simulink model "prve"  (Simulink 7.9)
settings: Solver=ode3  StartTime=0.0  StopTime=t_sim  RelTol=1e-3
values from neighbouring files (symbols this model uses):
  baud = 250000    [init.m]    (also in init_101_io_char_up_oloop.m)
  bulb = 100    [init.m]
  com = 'COM8'    [init.m]    (also in init_101_io_char_up_oloop.m = 'COM33')
  fan = 0    [init.m]
  fTf = 0.2    [init.m]    (also in init_101_io_char_up_oloop.m)
  fTl = 0.2    [init.m]    (also in init_101_io_char_up_oloop.m)
  fTt = 0.2    [init.m]    (also in init_101_io_char_up_oloop.m)
  LED = 0    [init.m]
  Ts = 0.1    [init.m]    (also in init_101_io_char_up_oloop.m)
libraries: tos_lib x1
settings Model: Creator=tom  LastModifiedBy=Katka
settings DataIOCC: LimitDataPoints=off
settings DebuggingCC: FcnCallInpInsideContextMsg=Use local settings  StrictBusMsg=Warning
settings GRTTargetCC: CombineOutputUpdateFcns=off  GRTInterface=on

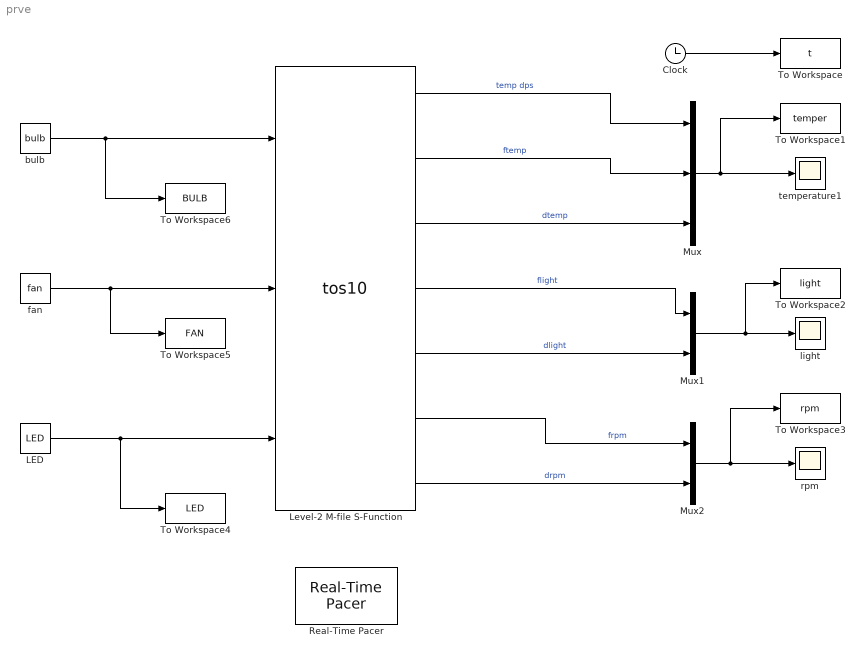
== system prve ==
  Clock : Clock
  LED : Constant  Value=LED
  Level-2 M-file S-Function : M-S-Function  FunctionName=tos10  Parameters=Ts,com,baud,fTt,fTl,fTf
  Mux : Mux  Inputs=3
  Mux1 : Mux  Inputs=2
  Mux2 : Mux  Inputs=2
  Real-Time Pacer : tos_lib/Real-Time Pacer  simTimePerRealTime=1
  To Workspace : ToWorkspace  VariableName=t  SampleTime=Ts
  To Workspace1 : ToWorkspace  VariableName=temper  SampleTime=Ts
  To Workspace2 : ToWorkspace  VariableName=light  SampleTime=Ts
  To Workspace3 : ToWorkspace  VariableName=rpm  SampleTime=Ts
  To Workspace4 : ToWorkspace  VariableName=LED  SampleTime=Ts
  To Workspace5 : ToWorkspace  VariableName=FAN  SampleTime=Ts
  To Workspace6 : ToWorkspace  VariableName=BULB  SampleTime=Ts
  bulb : Constant  Value=bulb
  fan : Constant  Value=fan
  light : Scope
      settings: YMax=85  MaxDataPoints=50000
  rpm : Scope
      settings: YMax=85  MaxDataPoints=50000
  temperature1 : Scope
      settings: TimeRange=2400  YMin=-2.5  YMax=45  SaveName=ScopeData4  MaxDataPoints=50000
  wires:
  bulb/1 -> Level-2 M-file S-Function/1, To Workspace6/1
  fan/1 -> Level-2 M-file S-Function/2, To Workspace5/1
  LED/1 -> Level-2 M-file S-Function/3, To Workspace4/1
  Mux/1 -> temperature1/1, To Workspace1/1
  Mux1/1 -> light/1, To Workspace2/1
  Clock/1 -> To Workspace/1
  Level-2 M-file S-Function/1 -> Mux/1  "temp dps"
  Level-2 M-file S-Function/2 -> Mux/2  "ftemp"
  Level-2 M-file S-Function/3 -> Mux/3  "dtemp"
  Level-2 M-file S-Function/4 -> Mux1/1  "flight"
  Level-2 M-file S-Function/5 -> Mux1/2  "dlight"
  Level-2 M-file S-Function/7 -> Mux2/2  "drpm"
  Mux2/1 -> To Workspace3/1, rpm/1
  Level-2 M-file S-Function/6 -> Mux2/1  "frpm"
